simulink model "Inverter_Ideal"  (R2018a)
settings: configuration reference "ModelConfig_var" (kept outside this file)
InitFcn:
  | %% BUS initialization
  | Xabc.A = 0;
  | Xabc.B = 0;
  | Xabc.C = 0;
  | % -------------------------------------------------------------------------
  | Simulink.Bus.createObject(Xabc)
  | XabcBus = slBus1;
  | clear slBus1
undefined symbols (not defined in the file): InputCircuit
settings Model: Creator=KIRTACA  LastModifiedBy=BEDNASA
settings ConfigSetRef: SourceLocation=Base Workspace

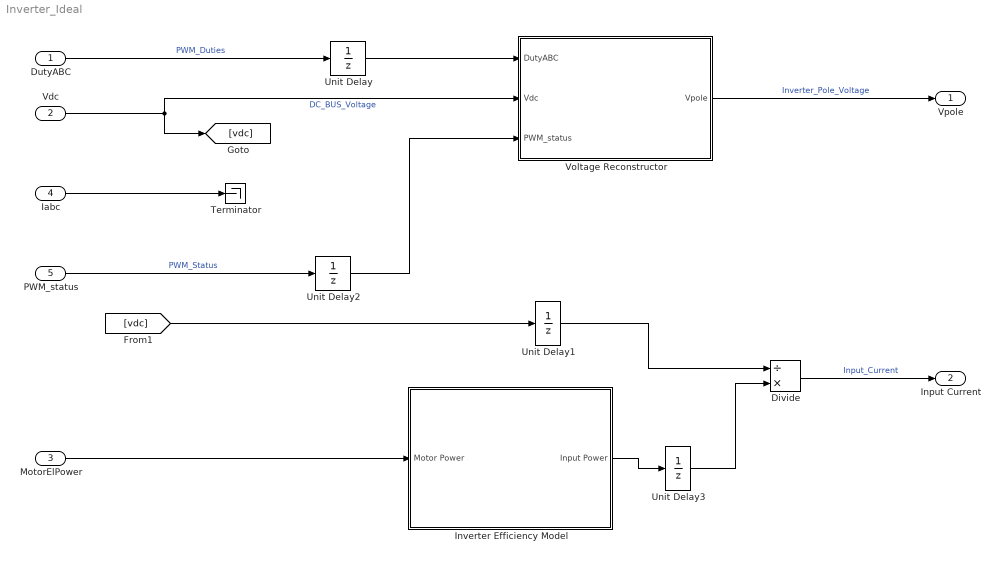
== system Inverter_Ideal ==
  DutyABC : Inport  OutDataTypeStr=Bus: XabcBus
  Vdc : Inport  Port=2
  MotorElPower : Inport  Port=3
  Iabc : Inport  Port=4  OutDataTypeStr=Bus: XabcBus
  PWM_status : Inport  Port=5
  Divide : Product  Inputs=/*
  Inverter Efficiency Model : Subsystem
  Terminator : Terminator
  Unit Delay : UnitDelay  SampleTime=-1
  Unit Delay1 : UnitDelay  InitialCondition=InputCircuit.Vdc_i  SampleTime=-1
  Unit Delay2 : UnitDelay  SampleTime=-1
  Unit Delay3 : UnitDelay  SampleTime=-1
  Voltage Reconstructor : MATLAB Function  TreatAsAtomicUnit=on
  "Vpole " : Outport  OutDataTypeStr=Bus: XabcBus
  Input Current : Outport  Port=2
  wires:
  Inverter Efficiency Model/1(Input Power) -> Unit Delay3/1
  Unit Delay3/1 -> Divide/2
  Unit Delay1/1 -> Divide/1
  [vdc] -> Unit Delay1/1
  DutyABC/1 -> Unit Delay/1  "PWM_Duties"
  Vdc/1 -> Voltage Reconstructor/2(Vdc), [vdc]  "DC_BUS_Voltage"
  MotorElPower/1 -> Inverter Efficiency Model/1(Motor Power)
  Divide/1 -> Input Current/1  "Input_Current"
  Voltage Reconstructor/1(Vpole) -> "Vpole "/1  "Inverter_Pole_Voltage"
  Iabc/1 -> Terminator/1
  PWM_status/1 -> Unit Delay2/1  "PWM_Status"
  Unit Delay/1 -> Voltage Reconstructor/1(DutyABC)
  Unit Delay2/1 -> Voltage Reconstructor/3(PWM_status)

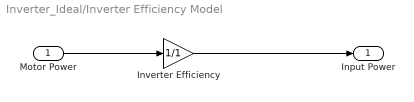
== system Inverter_Ideal/Inverter Efficiency Model ==
  Motor Power : Inport
  Inverter Efficiency : Gain  Gain=1/1
  Input Power : Outport
  wires:
  Motor Power/1 -> Inverter Efficiency/1
  Inverter Efficiency/1 -> Input Power/1

== matlab function Inverter_Ideal/Voltage Reconstructor ==
  data: DutyABC input Bus: XabcBus size=1; Vpole output Bus: XabcBus size=1; Vdc input; PWM_status input
function Vpole   = Vrec(DutyABC, Vdc, PWM_status)

if (PWM_status == 1)
    Da = DutyABC.A;
    Db = DutyABC.B;
    Dc = DutyABC.C;
else
    Da = 0.5;
    Db = 0.5;
    Dc = 0.5;
end
Vpole.A = Vdc * Da;
Vpole.B = Vdc * Db;
Vpole.C = Vdc * Dc;
